simulink model "motor_drive_model_mk20x2820x291"  (R2024a)
settings: Solver=FixedStepAuto  StartTime=0.0  StopTime=80  FixedStep=0.0001  MaxStep=0.1  RelTol=1e-3
undefined symbols (not defined in the file): batt_volt, gear_ratio, max_power, max_torque, motor_efficiency, wheel_radius
settings Model: Creator=shank  LastModifiedBy=Nitis
settings RTWCC: GPUComputeCapability=3.5

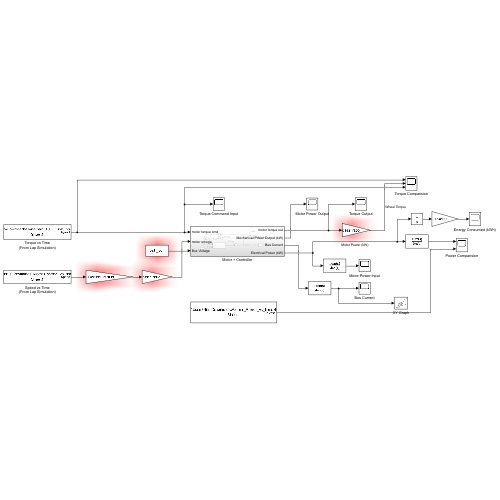
[thumbnail: Simulink's stored preview of the top-level diagram]
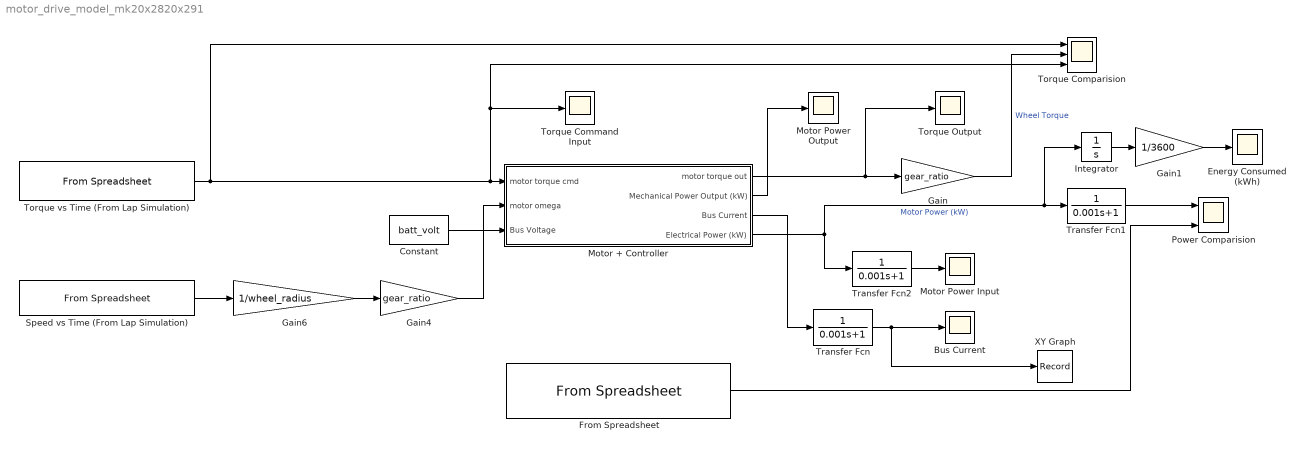
== system motor_drive_model_mk20x2820x291 ==
  Bus Current : Scope
  Constant : Constant  Value=batt_volt
  Energy Consumed (kWh) : Scope
  From Spreadsheet : FromSpreadsheet  FileName=C:\Users\Nitis\Downloads\Aromal_Power_vs_time.xlsx  ExtrapolationBeforeFirstDataPoint=Ground value  ExtrapolationAfterLastDataPoint=Ground value
  Gain : Gain  Gain=gear_ratio
  Gain1 : Gain  Gain=1/3600
  Gain4 : Gain  Gain=gear_ratio
  Gain6 : Gain  Gain=1/wheel_radius
  Integrator : Integrator
  Motor + Controller : Subsystem
  Motor Power Input : Scope
  Motor Power Output : Scope
  Power Comparision : Scope  NumInputPorts=2
  Speed vs Time (From Lap Simulation) : FromSpreadsheet  FileName=C:\Users\Nitis\Downloads\Aromal_speed_vs_time (1).xlsx  Range=A1:B9750  ExtrapolationBeforeFirstDataPoint=Ground value  ExtrapolationAfterLastDataPoint=Ground value
  Torque Command Input : Scope
  Torque Comparision : Scope  NumInputPorts=3
  Torque Output : Scope
  Torque vs Time (From Lap Simulation) : FromSpreadsheet  FileName=C:\Users\Nitis\Downloads\JonathanLTS_-_Time_vs_Torque.xlsx  Range=A1:B9750  ExtrapolationBeforeFirstDataPoint=Ground value  ExtrapolationAfterLastDataPoint=Ground value
  Transfer Fcn : TransferFcn  Denominator=[0.001 1]
  Transfer Fcn1 : TransferFcn  Denominator=[0.001 1]
  Transfer Fcn2 : TransferFcn  Denominator=[0.001 1]
  XY Graph : Record  Filename=bus current.xlsx  FileSettingsInternal="{\"entries\":[{\"content\":{\"excelSettings\":{\"content\":{},\"type\":\"Streamout.ExcelSettings\"}},\"type\":\"Streamout.FileSettingStorage\",\"uuid\":\"\"}],\"packageUris\":[\"http:\\/\\/schema.mathworks.com\\/mf0\\/streamout_blocks\\/R2020a\"],\"version\":\"1.0\"}"  Layout=[1 1]  SignalsInternal="{\"entries\":[{\"content\":{\"signals\":[{\"content\":{\"blockPath\":[],\"dimensions\":[1],\"domain\":\"\",\"lineColor\":\"#0072bd\",\"plots\":[ 1 ],\"port\":1,\"signalID\":1,\"signalName\":\"Transfer Fcn\"},\"type\":\"RecordBlkView.Signal\",\"uuid\":\"\"}]},\"type\":\"RecordBlkView.InputSignals\",\"uuid\":\"\"}],\"packageUris\":[\"http:\\/\\/schema.mathworks.com\\/mf0\\/streamout_blocks\\/R2020a\"],\"version\":\"1.0\"}"  CompatibilityTag=XY
  wires:
  Torque vs Time (From Lap Simulation)/1 -> Torque Comparision/1, Torque Comparision/3, Torque Command Input/1, Motor + Controller/1(motor torque cmd)
  Constant/1 -> Motor + Controller/3(Bus Voltage)
  Motor + Controller/4(Electrical Power (kW)) -> Transfer Fcn2/1, Transfer Fcn1/1, Integrator/1  "Motor Power (kW)"
  Motor + Controller/3(Bus Current) -> Transfer Fcn/1
  Gain/1 -> Torque Comparision/2  "Wheel Torque"
  Gain6/1 -> Gain4/1
  Gain4/1 -> Motor + Controller/2(motor omega)
  Speed vs Time (From Lap Simulation)/1 -> Gain6/1
  Integrator/1 -> Gain1/1
  From Spreadsheet/1 -> Power Comparision/2
  Motor + Controller/1(motor torque out) -> Gain/1, Torque Output/1
  Motor + Controller/2(Mechanical Power Output (kW)) -> Motor Power Output/1
  Gain1/1 -> Energy Consumed (kWh)/1
  Transfer Fcn/1 -> XY Graph/1, Bus Current/1
  Transfer Fcn1/1 -> Power Comparision/1
  Transfer Fcn2/1 -> Motor Power Input/1

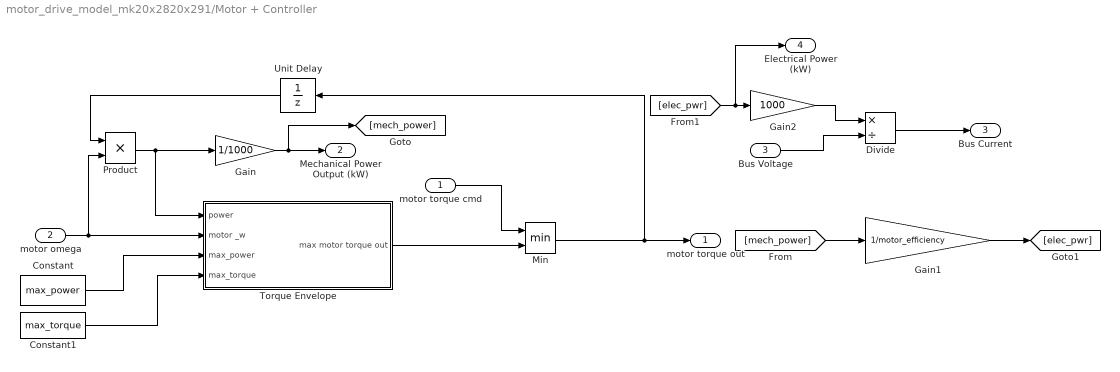
== system motor_drive_model_mk20x2820x291/Motor + Controller ==
  motor torque cmd : Inport
  motor omega : Inport  Port=2
  Bus Voltage : Inport  Port=3
  Constant : Constant  Value=max_power
  Constant1 : Constant  Value=max_torque
  Divide : Product  Inputs=*/
  Gain : Gain  Gain=1/1000
  Gain1 : Gain  Gain=1/motor_efficiency
  Gain2 : Gain  Gain=1000
  Min : MinMax  Inputs=2
  Product : Product
  Torque Envelope : Subsystem
  Unit Delay : UnitDelay  SampleTime=-1  HasFrameUpgradeWarning=on
  motor torque out : Outport
  Mechanical Power Output (kW) : Outport  Port=2
  Bus Current : Outport  Port=3
  Electrical Power (kW) : Outport  Port=4
  wires:
  Gain/1 -> Mechanical Power Output (kW)/1, [mech_power]
  motor torque cmd/1 -> Min/1
  Unit Delay/1 -> Product/1
  Constant1/1 -> Torque Envelope/4(max_torque)
  Divide/1 -> Bus Current/1
  motor omega/1 -> Product/2, Torque Envelope/2(motor _w)
  Torque Envelope/1(max motor torque out) -> Min/2
  Bus Voltage/1 -> Divide/2
  Gain1/1 -> [elec_pwr]
  [mech_power] -> Gain1/1
  Product/1 -> Torque Envelope/1(power), Gain/1
  Constant/1 -> Torque Envelope/3(max_power)
  [elec_pwr] -> Electrical Power (kW)/1, Gain2/1
  Gain2/1 -> Divide/1
  Min/1 -> Unit Delay/1, motor torque out/1

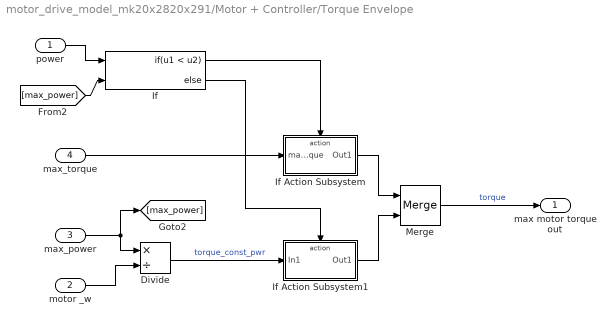
== system motor_drive_model_mk20x2820x291/Motor + Controller/Torque Envelope ==
  power : Inport
  motor _w : Inport  Port=2
  max_power : Inport  Port=3
  max_torque : Inport  Port=4
  Divide : Product  Inputs=*/
  If : If  NumInputs=2  IfExpression=u1 < u2
  If Action Subsystem : Subsystem  TreatAsAtomicUnit=on
  If Action Subsystem1 : Subsystem  TreatAsAtomicUnit=on
  Merge : Merge
  max motor torque out : Outport
  wires:
  max_torque/1 -> If Action Subsystem/1(max_torque)
  If/1 -> If Action Subsystem/Action
  max_power/1 -> [max_power], Divide/1
  If Action Subsystem1/1(Out1) -> Merge/2
  Divide/1 -> If Action Subsystem1/1(In1)  "torque_const_pwr"
  If Action Subsystem/1(Out1) -> Merge/1
  If/2 -> If Action Subsystem1/Action
  [max_power] -> If/2
  power/1 -> If/1
  Merge/1 -> max motor torque out/1  "torque"
  motor _w/1 -> Divide/2

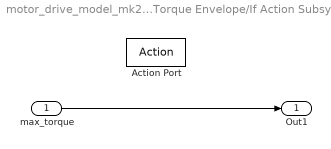
== system motor_drive_model_mk20x2820x291/Motor + Controller/Torque Envelope/If Action Subsystem ==
  max_torque : Inport
  Action Port : ActionPort  ActionPortLabel=if(u1 < u2)
  Out1 : Outport
  wires:
  max_torque/1 -> Out1/1

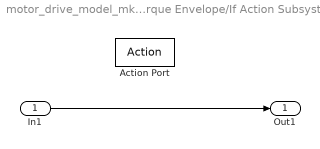
== system motor_drive_model_mk20x2820x291/Motor + Controller/Torque Envelope/If Action Subsystem1 ==
  In1 : Inport
  Action Port : ActionPort  ActionPortLabel=else
  Out1 : Outport
  wires:
  In1/1 -> Out1/1
